simulink model "circuit1"  (R2015b)
settings: Solver=VariableStepAuto  StartTime=0.0  StopTime=0.25  RelTol=1e-3
values from neighbouring files (symbols this model uses):
  C = 1e-6    (= 1e-06)    [l3_1.m]
  L = 20    [l3_1.m]
  R = 1e3    (= 1000)    [l3_1.m]
settings Model: Creator=ovi  LastModifiedBy=ovi

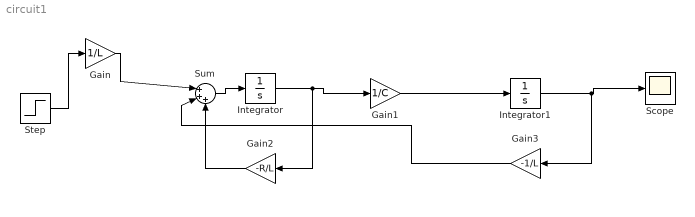
== system circuit1 ==
  Gain : Gain  Gain=1/L
  Gain1 : Gain  Gain=1/C
  Gain2 : Gain  Gain=-R/L
  Gain3 : Gain  Gain=-1/L
  Integrator : Integrator
  Integrator1 : Integrator
  Scope : Scope
  Step : Step  Time=0.0  SampleTime=0
  Sum : Sum  Inputs=|+++
  wires:
  Step/1 -> Gain/1
  Gain/1 -> Sum/1
  Sum/1 -> Integrator/1
  Integrator/1 -> Gain2/1, Gain1/1
  Gain1/1 -> Integrator1/1
  Gain2/1 -> Sum/3
  Integrator1/1 -> Gain3/1, Scope/1
  Gain3/1 -> Sum/2
